simulink model "bus_as_currentsource_charging_discharging_battery_1"  (R2023a)
settings: Solver=VariableStepAuto  StartTime=0.0  StopTime=0.01  RelTol=1e-3
libraries: spsParallelRLCBranchLib x72, spsCurrentMeasurementLib x27, spsVoltageMeasurementLib x27, spspowerguiLib x25, spsControlledVoltageSourceLib x24, spsVariableResistorLib x24, spsSeriesRLCBranchLib x6, spsMosfetLib x2, sdolib x1, spsControlledCurrentSourceLib x1, spsGroundLib x1
(part 1 of 4)
settings Model: Creator=mluser  LastModifiedBy=Amith

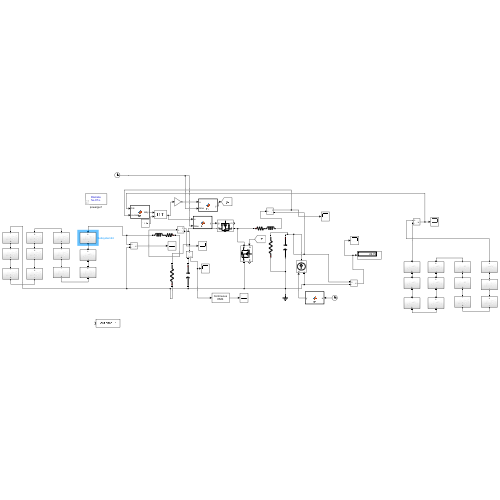
[thumbnail: Simulink's stored preview of the top-level diagram]
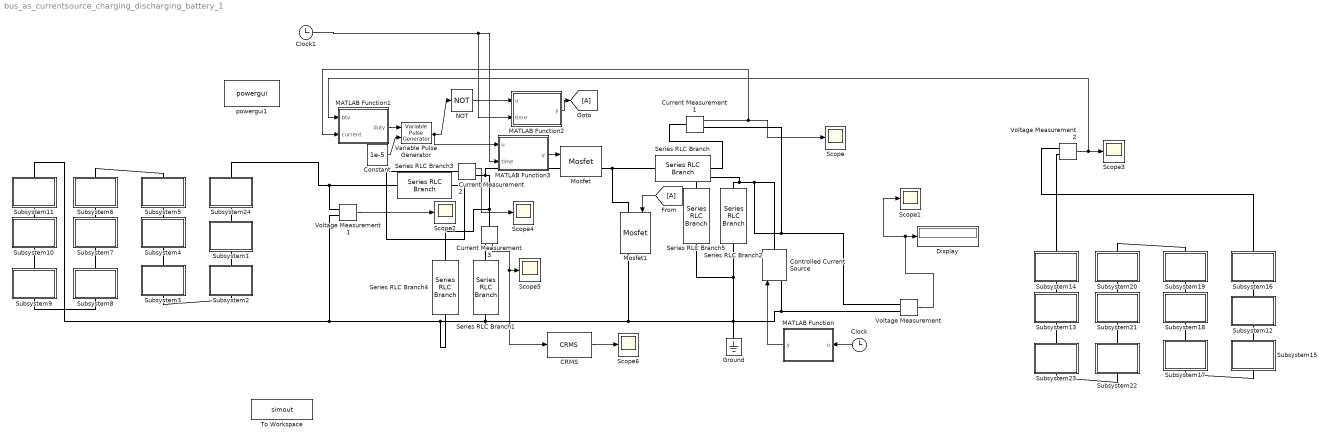
== system bus_as_currentsource_charging_discharging_battery_1 ==
  CRMS : sdolib/RMS Blocks/CRMS
  Clock : Clock
  Clock1 : Clock
  Constant : Constant  Value=1e-5
  Controlled Current Source : spsControlledCurrentSourceLib/Controlled Current Source  Initialize=on  Source_Type=AC  Amplitude=0  Phase=0  Frequency=0  Measurements=None
  Current Measurement1 : spsCurrentMeasurementLib/Current Measurement  PhasorSimulation=off  OutputType=Complex  PSBequivalent=0
  Current Measurement2 : spsCurrentMeasurementLib/Current Measurement  PhasorSimulation=off  OutputType=Complex  PSBequivalent=0
  Current Measurement3 : spsCurrentMeasurementLib/Current Measurement  PhasorSimulation=off  OutputType=Complex  PSBequivalent=0
  Display : Display
  From : From
  Goto : Goto
  Ground : spsGroundLib/Ground  LConnTagsString=a
  MATLAB Function : MATLAB Function  TreatAsAtomicUnit=on
  MATLAB Function1 : MATLAB Function  TreatAsAtomicUnit=on
  MATLAB Function2 : MATLAB Function  TreatAsAtomicUnit=on
  MATLAB Function3 : MATLAB Function  TreatAsAtomicUnit=on
  Mosfet : spsMosfetLib/Mosfet  Ron=0.1  Lon=0  Rd=0.01  Vfd=0  IC=0  Rs=1e5  Cs=inf  Measurements=on
  Mosfet1 : spsMosfetLib/Mosfet  Ron=0.1  Lon=0  Rd=0.01  Vfd=0  IC=0  Rs=1e5  Cs=inf  Measurements=on
  NOT : Logic  Operator=NOT  IconShape=distinctive  AllPortsSameDT=off  OutDataTypeStr=boolean
  Scope{,1..6} (7 alike) : Scope
  Series RLC Branch : spsSeriesRLCBranchLib/Series RLC Branch  LConnTagsString=__new0  RConnTagsString=__new0  BranchType=RL  Resistance=2.4e-3  Inductance=22e-6  SetiL0=off  InitialCurrent=0  Capacitance=1e-6  Setx0=off  InitialVoltage=0  Measurements=None
  Series RLC Branch1 : spsSeriesRLCBranchLib/Series RLC Branch  LConnTagsString=__new0  RConnTagsString=__new0  BranchType=C  Resistance=1  Inductance=1e-3  SetiL0=off  InitialCurrent=0  Capacitance=94e-6  Setx0=off  InitialVoltage=0  Measurements=None
  Series RLC Branch2 : spsSeriesRLCBranchLib/Series RLC Branch  LConnTagsString=__new0  RConnTagsString=__new0  BranchType=C  Resistance=1  Inductance=1e-3  SetiL0=off  InitialCurrent=0  Capacitance=188e-6  Setx0=off  InitialVoltage=0  Measurements=None
  Series RLC Branch3 : spsSeriesRLCBranchLib/Series RLC Branch  LConnTagsString=__new0  RConnTagsString=__new0  BranchType=RL  Resistance=2.4e-3  Inductance=22e-6  SetiL0=off  InitialCurrent=0  Capacitance=256.86e-6  Setx0=off  InitialVoltage=0  Measurements=None
  Series RLC Branch4 : spsSeriesRLCBranchLib/Series RLC Branch  LConnTagsString=__new0  RConnTagsString=__new0  BranchType=R  Resistance=10e3  Inductance=22e-6  SetiL0=off  InitialCurrent=0  Capacitance=256.86e-6  Setx0=off  InitialVoltage=0  Measurements=None
  Series RLC Branch5 : spsSeriesRLCBranchLib/Series RLC Branch  LConnTagsString=__new0  RConnTagsString=__new0  BranchType=R  Resistance=10e3  Inductance=22e-6  SetiL0=off  InitialCurrent=0  Capacitance=256.86e-6  Setx0=off  InitialVoltage=0  Measurements=None
  Subsystem1 : Subsystem
  Subsystem10 : Subsystem
  Subsystem11 : Subsystem
  Subsystem12 : Subsystem
  Subsystem13 : Subsystem
  Subsystem14 : Subsystem
  Subsystem15 : Subsystem
  Subsystem16 : Subsystem
  Subsystem17 : Subsystem
  Subsystem18 : Subsystem
  Subsystem19 : Subsystem
  Subsystem2 : Subsystem
  Subsystem20 : Subsystem
  Subsystem21 : Subsystem
  Subsystem22 : Subsystem
  Subsystem23 : Subsystem
  Subsystem24 : Subsystem
  Subsystem3 : Subsystem
  Subsystem4 : Subsystem
  Subsystem5 : Subsystem
  Subsystem6 : Subsystem
  Subsystem7 : Subsystem
  Subsystem8 : Subsystem
  Subsystem9 : Subsystem
  To Workspace : ToWorkspace  VariableName=simout  SaveFormat=Timeseries  SampleTime=-1
  Variable Pulse Generator : VariablePulseGenerator  SampleTime=0.1
  Voltage Measurement : spsVoltageMeasurementLib/Voltage Measurement  PhasorSimulation=off  OutputType=Complex  PSBequivalent=0
  Voltage Measurement1 : spsVoltageMeasurementLib/Voltage Measurement  PhasorSimulation=off  OutputType=Complex  PSBequivalent=0
  Voltage Measurement2 : spsVoltageMeasurementLib/Voltage Measurement  PhasorSimulation=off  OutputType=Complex  PSBequivalent=0
  powergui1 : spspowerguiLib/powergui  Priority=1  SimulationMode=Discrete  SampleTime=5e-7  frequency=60  Iterations=50  frequencyindice=0  Pbase=100e6  ErrMax=1e-4  UnitsV=kV  UnitsW=MW  buscounter=0  FunctionMessages=off  echomessages=off  EnableUseOfTLC=off  CurrentSourceSwitches=off  DisableSnubberDevices=off  DisableRonSwitches=off  DisableVfSwitches=off  DisplayEquations=off  AutomaticDiscreteSolvers=off  SolverType=Tustin/Backward Euler (TBE)  Interpol=off  ExternalGateDelay=off  methode=off  Ts=100  x0status=blocks  SPID=on  SwTol=0  HookPort=off  NonlinearTolerance=1e-4  nMaxIteration=100  ContinueOnMaxIteration=off  RestoreLinks=warning  ResistiveCurrentMeasurement=off  Frange=[0:2:500]  Ylog=off  Xlog=on  ShowGrid=off  save=off  variable=ZData  structure=0  ZoomFFT=off  StartTime=0.0  cycles=1  DisplayStyle=1  fundamental=60  FreqAxis=off  MaxFrequency=1000  frequencyindicesteady=1  RmsSteady=1  display=off
  wires:
  Clock1/1 -> MATLAB Function3/2(time), MATLAB Function2/2(time)
  Variable Pulse Generator/1 -> MATLAB Function3/1(u), NOT/1
  MATLAB Function1/1(duty) -> Variable Pulse Generator/1
  Current Measurement2/1 -> Scope4/1
  MATLAB Function/1(y) -> Controlled Current Source/1
  MATLAB Function3/1(y) -> Mosfet/1
  From/1 -> Mosfet1/1
  Voltage Measurement1/1 -> Scope2/1
  Clock/1 -> MATLAB Function/1(u)
  NOT/1 -> MATLAB Function2/1(u)
  Voltage Measurement2/1 -> MATLAB Function1/1(btv), Scope3/1
  Current Measurement1/1 -> MATLAB Function1/2(current), Scope/1
  MATLAB Function2/1(y) -> Goto/1
  Current Measurement3/1 -> CRMS/1, Scope5/1
  Constant/1 -> Variable Pulse Generator/2
  Voltage Measurement/1 -> Scope1/1, Display/1
  CRMS/1 -> Scope6/1
  connections:
  Mosfet/LConn1 -- Current Measurement2/RConn1 -- Series RLC Branch4/RConn1 -- Current Measurement3/LConn1
  Voltage Measurement/LConn2 -- Ground/LConn1 -- Series RLC Branch5/LConn1 -- Series RLC Branch2/RConn1 -- Subsystem11/LConn1 -- Voltage Measurement1/LConn2 -- Series RLC Branch4/LConn1 -- Series RLC Branch1/RConn1 -- Mosfet1/RConn1 -- Controlled Current Source/LConn1
  Voltage Measurement/LConn1 -- Controlled Current Source/RConn1 -- Series RLC Branch5/RConn1 -- Series RLC Branch2/LConn1 -- Current Measurement1/RConn1
  Mosfet1/LConn1 -- Series RLC Branch/LConn1 -- Mosfet/RConn1
  Voltage Measurement1/LConn1 -- Subsystem24/RConn1 -- Series RLC Branch3/RConn1
  Series RLC Branch1/LConn1 -- Current Measurement3/RConn1
  Current Measurement2/LConn1 -- Series RLC Branch3/LConn1
  Current Measurement1/LConn1 -- Series RLC Branch/RConn1
  Subsystem1/RConn1 -- Subsystem24/LConn1
  Subsystem2/RConn1 -- Subsystem1/LConn1
  Subsystem3/RConn1 -- Subsystem2/LConn1
  Subsystem6/RConn1 -- Subsystem5/LConn1
  Subsystem5/RConn1 -- Subsystem4/LConn1
  Subsystem10/RConn1 -- Subsystem9/LConn1
  Subsystem4/RConn1 -- Subsystem3/LConn1
  Subsystem7/RConn1 -- Subsystem6/LConn1
  Subsystem8/LConn1 -- Subsystem9/RConn1
  Subsystem11/RConn1 -- Subsystem10/LConn1
  Subsystem8/RConn1 -- Subsystem7/LConn1
  Subsystem12/RConn1 -- Subsystem16/LConn1
  Subsystem22/RConn1 -- Subsystem21/LConn1
  Subsystem20/RConn1 -- Subsystem19/LConn1
  Subsystem14/RConn1 -- Subsystem13/LConn1
  Subsystem21/RConn1 -- Subsystem20/LConn1
  Subsystem15/RConn1 -- Subsystem12/LConn1
  Subsystem19/RConn1 -- Subsystem18/LConn1
  Subsystem13/RConn1 -- Subsystem23/LConn1
  Subsystem18/RConn1 -- Subsystem17/LConn1
  Subsystem14/LConn1 -- Voltage Measurement2/LConn2
  Subsystem16/RConn1 -- Voltage Measurement2/LConn1
  Subsystem15/LConn1 -- Subsystem17/RConn1
  Subsystem22/LConn1 -- Subsystem23/RConn1

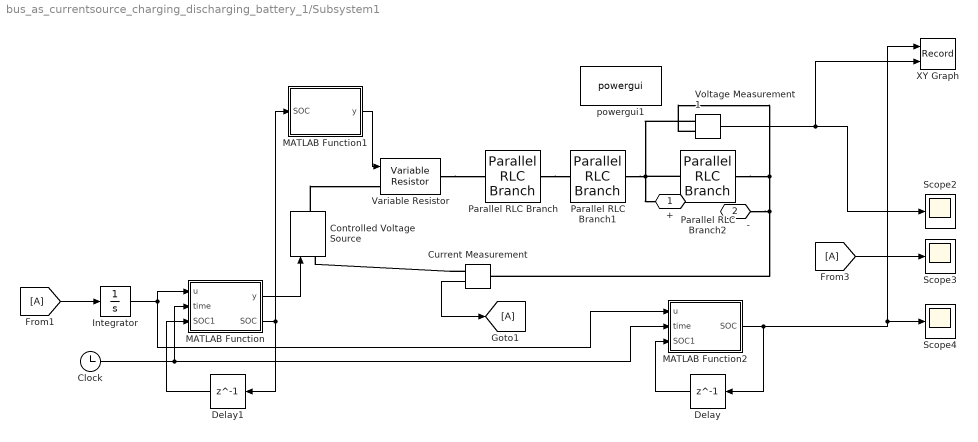
== system bus_as_currentsource_charging_discharging_battery_1/Subsystem1 ==
  Clock : Clock
  Controlled Voltage Source : spsControlledVoltageSourceLib/Controlled Voltage Source  Initialize=on  Source_Type=DC  Amplitude=0  Phase=0  Frequency=0  Measurements=None
  Current Measurement : spsCurrentMeasurementLib/Current Measurement  PhasorSimulation=off  OutputType=Complex  PSBequivalent=0
  Delay : Delay  DelayLength=1  InitialCondition=0
  Delay1 : Delay  DelayLength=1  InitialCondition=0
  From1 : From
  From3 : From
  Goto1 : Goto
  Integrator : Integrator
  MATLAB Function : MATLAB Function  TreatAsAtomicUnit=on
  MATLAB Function1 : MATLAB Function  TreatAsAtomicUnit=on
  MATLAB Function2 : MATLAB Function  TreatAsAtomicUnit=on
  Parallel RLC Branch : spsParallelRLCBranchLib/Parallel RLC Branch  LConnTagsString=a  RConnTagsString=__new0  BranchType=RC  Resistance=15.5e-3  Inductance=1e-3  SetiL0=off  InitialCurrent=0  Capacitance=1028.7  Setx0=off  InitialVoltage=0  Measurements=None
  Parallel RLC Branch1 : spsParallelRLCBranchLib/Parallel RLC Branch  LConnTagsString=a  RConnTagsString=__new0  BranchType=RC  Resistance=18.3e-3  Inductance=1e-3  SetiL0=off  InitialCurrent=0  Capacitance=5756.6  Setx0=off  InitialVoltage=0  Measurements=None
  Parallel RLC Branch2 : spsParallelRLCBranchLib/Parallel RLC Branch  LConnTagsString=a  RConnTagsString=__new0  BranchType=R  Resistance=1e9  Inductance=1e-3  SetiL0=off  InitialCurrent=0  Capacitance=5756.6  Setx0=off  InitialVoltage=0  Measurements=None
  Scope2 : Scope
  Scope3 : Scope
  Scope4 : Scope
  Variable Resistor : spsVariableResistorLib/Variable Resistor  Rabsmin=1e-3
      settings: LibrarySourceBlock=sps_lib/Passives/Variable Resistor
  Voltage Measurement1 : spsVoltageMeasurementLib/Voltage Measurement  PhasorSimulation=off  OutputType=Complex  PSBequivalent=0
  XY Graph : Record  FileSettingsInternal="{\"entries\":[{\"content\":{\"excelSettings\":{\"content\":{},\"type\":\"Streamout.ExcelSettings\"}},\"type\":\"Streamout.FileSettingStorage\",\"uuid\":\"4061d31d-d8a3-4fd0-9d33-75a5776b2999\"}],\"packageUris\":[\"http://schema.mathworks.com/mf0/streamout_blocks/R2020a\"],\"version\":\"1.0\"}"  Layout=[1 1]  SignalsInternal="{\"entries\":[{\"content\":{\"signals\":[{\"content\":{\"blockPath\":[\"bus_as_currentsource_charging_discharging_battery_1/Subsystem1/XY Graph\"],\"dimensions\":[1],\"domain\":\"bus_as_currentsource_charging_discharging_battery_1/Subsystem1/XY Graph\",\"lineColor\":\"#a2142f\",\"port\":1,\"sid\":[\"\"],\"signalID\":203,\"signalName\":\"MATLAB Function2\"},\"type\":\"RecordBlkView.Signal\",\"uuid\":\"0f566fc9-80d1-47d5-bf49-5749430e9d0a\"},{\"content\":{\"blockPath\":[\"bus_as_currentsource_charging_discharging_battery_1/Subsystem1/XY Graph\"],\"dimensions\":[1],\"domain\":\"bus_as_currentsource_charging_discharging_battery_1/Subsystem1/XY Graph\",\"lineColor\":\"#139fff\",\"port\":2,\"sid\":[\"\"],\"signalID\":207,\"signalName\":\"Voltage Measurement1\"},\"type\":\"RecordBlkView.Signal\",\"uuid\":\"ed6d931e-a948-4cdc-a839-bfb3bbb69890\"}]},\"type\":\"RecordBlkView.InputSignals\",\"uuid\":\"04ab3669-a145-4f40-a759-cdf575706550\"}],\"packageUris\":[\"http://schema.mathworks.com/mf0/streamout_blocks/R2020a\"],\"version\":\"1.0\"}"  VisualizationBindings="{\"xyplotplugin\":{\"info\":[{\"series\":[],\"subplotID\":1}]}}"  CompatibilityTag=XY
  powergui1 : spspowerguiLib/powergui  Priority=1  SimulationMode=Discrete  SampleTime=2e-7  frequency=60  Iterations=50  frequencyindice=0  Pbase=100e6  ErrMax=1e-4  UnitsV=kV  UnitsW=MW  buscounter=0  FunctionMessages=off  echomessages=off  EnableUseOfTLC=off  CurrentSourceSwitches=off  DisableSnubberDevices=off  DisableRonSwitches=off  DisableVfSwitches=off  DisplayEquations=off  AutomaticDiscreteSolvers=off  SolverType=Tustin/Backward Euler (TBE)  Interpol=off  ExternalGateDelay=off  methode=off  Ts=100  x0status=blocks  SPID=on  SwTol=0  HookPort=off  NonlinearTolerance=1e-4  nMaxIteration=100  ContinueOnMaxIteration=off  RestoreLinks=warning  ResistiveCurrentMeasurement=off  Frange=[0:2:500]  Ylog=off  Xlog=on  ShowGrid=off  save=off  variable=ZData  structure=0  ZoomFFT=off  StartTime=0.0  cycles=1  DisplayStyle=1  fundamental=60  FreqAxis=off  MaxFrequency=1000  frequencyindicesteady=1  RmsSteady=1  display=off
  + : PMIOPort  Side=Right
  - : PMIOPort  Port=2  Side=Left
  wires:
  Current Measurement/1 -> Goto1/1
  From3/1 -> Scope3/1
  Voltage Measurement1/1 -> XY Graph/2, Scope2/1
  MATLAB Function2/1(SOC) -> Delay/1, XY Graph/1, Scope4/1
  From1/1 -> Integrator/1
  MATLAB Function/1(y) -> Controlled Voltage Source/1
  MATLAB Function1/1(y) -> Variable Resistor/1
  Integrator/1 -> MATLAB Function2/1(u), MATLAB Function/1(u)
  Clock/1 -> MATLAB Function2/2(time), MATLAB Function/2(time)
  MATLAB Function/2(SOC) -> Delay1/1, MATLAB Function1/1(SOC)
  Delay/1 -> MATLAB Function2/3(SOC1)
  Delay1/1 -> MATLAB Function/3(SOC1)
  connections:
  Variable Resistor/RConn1 -- Parallel RLC Branch/LConn1
  Parallel RLC Branch1/RConn1 -- Parallel RLC Branch2/LConn1 -- +/RConn1 -- Voltage Measurement1/LConn1
  Voltage Measurement1/LConn2 -- Parallel RLC Branch2/RConn1 -- -/RConn1 -- Current Measurement/LConn1
  Controlled Voltage Source/RConn1 -- Variable Resistor/LConn1
  Current Measurement/RConn1 -- Controlled Voltage Source/LConn1
  Parallel RLC Branch/RConn1 -- Parallel RLC Branch1/LConn1

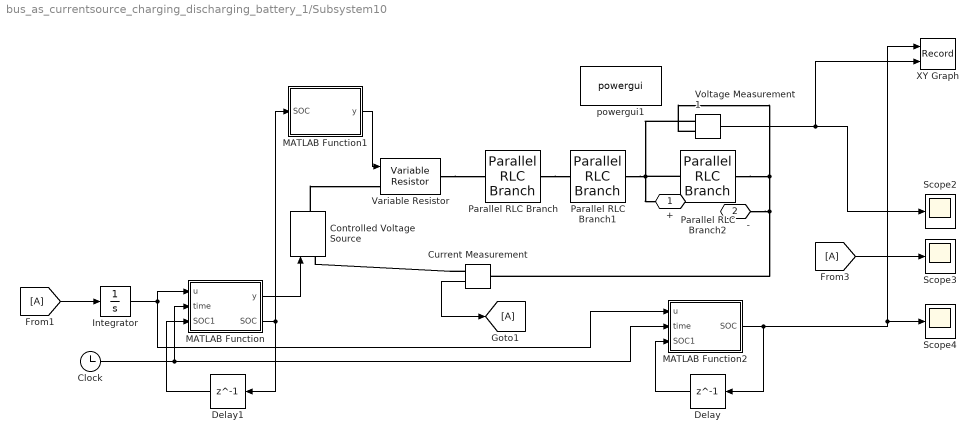
== system bus_as_currentsource_charging_discharging_battery_1/Subsystem10 ==
  Clock : Clock
  Controlled Voltage Source : spsControlledVoltageSourceLib/Controlled Voltage Source  Initialize=on  Source_Type=DC  Amplitude=0  Phase=0  Frequency=0  Measurements=None
  Current Measurement : spsCurrentMeasurementLib/Current Measurement  PhasorSimulation=off  OutputType=Complex  PSBequivalent=0
  Delay : Delay  DelayLength=1  InitialCondition=0
  Delay1 : Delay  DelayLength=1  InitialCondition=0
  From1 : From
  From3 : From
  Goto1 : Goto
  Integrator : Integrator
  MATLAB Function : MATLAB Function  TreatAsAtomicUnit=on
  MATLAB Function1 : MATLAB Function  TreatAsAtomicUnit=on
  MATLAB Function2 : MATLAB Function  TreatAsAtomicUnit=on
  Parallel RLC Branch : spsParallelRLCBranchLib/Parallel RLC Branch  LConnTagsString=a  RConnTagsString=__new0  BranchType=RC  Resistance=15.5e-3  Inductance=1e-3  SetiL0=off  InitialCurrent=0  Capacitance=1028.7  Setx0=off  InitialVoltage=0  Measurements=None
  Parallel RLC Branch1 : spsParallelRLCBranchLib/Parallel RLC Branch  LConnTagsString=a  RConnTagsString=__new0  BranchType=RC  Resistance=18.3e-3  Inductance=1e-3  SetiL0=off  InitialCurrent=0  Capacitance=5756.6  Setx0=off  InitialVoltage=0  Measurements=None
  Parallel RLC Branch2 : spsParallelRLCBranchLib/Parallel RLC Branch  LConnTagsString=a  RConnTagsString=__new0  BranchType=R  Resistance=1e9  Inductance=1e-3  SetiL0=off  InitialCurrent=0  Capacitance=5756.6  Setx0=off  InitialVoltage=0  Measurements=None
  Scope2 : Scope
  Scope3 : Scope
  Scope4 : Scope
  Variable Resistor : spsVariableResistorLib/Variable Resistor  Rabsmin=1e-3
      settings: LibrarySourceBlock=sps_lib/Passives/Variable Resistor
  Voltage Measurement1 : spsVoltageMeasurementLib/Voltage Measurement  PhasorSimulation=off  OutputType=Complex  PSBequivalent=0
  XY Graph : Record  FileSettingsInternal="{\"entries\":[{\"content\":{\"excelSettings\":{\"content\":{},\"type\":\"Streamout.ExcelSettings\"}},\"type\":\"Streamout.FileSettingStorage\",\"uuid\":\"1acef1d3-1533-4111-95e4-15d755019280\"}],\"packageUris\":[\"http://schema.mathworks.com/mf0/streamout_blocks/R2020a\"],\"version\":\"1.0\"}"  Layout=[1 1]  SignalsInternal="{\"entries\":[{\"content\":{\"signals\":[{\"content\":{\"blockPath\":[\"bus_as_currentsource_charging_discharging_battery_1/Subsystem10/XY Graph\"],\"dimensions\":[1],\"domain\":\"bus_as_currentsource_charging_discharging_battery_1/Subsystem10/XY Graph\",\"lineColor\":\"#ff6929\",\"port\":1,\"sid\":[\"\"],\"signalID\":211,\"signalName\":\"MATLAB Function2\"},\"type\":\"RecordBlkView.Signal\",\"uuid\":\"1c5f61ff-3524-492e-ac01-ee5e6fde95d9\"},{\"content\":{\"blockPath\":[\"bus_as_currentsource_charging_discharging_battery_1/Subsystem10/XY Graph\"],\"dimensions\":[1],\"domain\":\"bus_as_currentsource_charging_discharging_battery_1/Subsystem10/XY Graph\",\"lineColor\":\"#b746ff\",\"port\":2,\"sid\":[\"\"],\"signalID\":215,\"signalName\":\"Voltage Measurement1\"},\"type\":\"RecordBlkView.Signal\",\"uuid\":\"4a662dbb-6ada-419c-879e-f8766603ed58\"}]},\"type\":\"RecordBlkView.InputSignals\",\"uuid\":\"1ce9e898-f152-4a36-91f2-a929c2b13ee4\"}],\"packageUris\":[\"http://schema.mathworks.com/mf0/streamout_blocks/R2020a\"],\"version\":\"1.0\"}"  VisualizationBindings="{\"xyplotplugin\":{\"info\":[{\"series\":[],\"subplotID\":1}]}}"  CompatibilityTag=XY
  powergui1 : spspowerguiLib/powergui  Priority=1  SimulationMode=Discrete  SampleTime=2e-7  frequency=60  Iterations=50  frequencyindice=0  Pbase=100e6  ErrMax=1e-4  UnitsV=kV  UnitsW=MW  buscounter=0  FunctionMessages=off  echomessages=off  EnableUseOfTLC=off  CurrentSourceSwitches=off  DisableSnubberDevices=off  DisableRonSwitches=off  DisableVfSwitches=off  DisplayEquations=off  AutomaticDiscreteSolvers=off  SolverType=Tustin/Backward Euler (TBE)  Interpol=off  ExternalGateDelay=off  methode=off  Ts=100  x0status=blocks  SPID=on  SwTol=0  HookPort=off  NonlinearTolerance=1e-4  nMaxIteration=100  ContinueOnMaxIteration=off  RestoreLinks=warning  ResistiveCurrentMeasurement=off  Frange=[0:2:500]  Ylog=off  Xlog=on  ShowGrid=off  save=off  variable=ZData  structure=0  ZoomFFT=off  StartTime=0.0  cycles=1  DisplayStyle=1  fundamental=60  FreqAxis=off  MaxFrequency=1000  frequencyindicesteady=1  RmsSteady=1  display=off
  + : PMIOPort  Side=Right
  - : PMIOPort  Port=2  Side=Left
  wires:
  Current Measurement/1 -> Goto1/1
  From3/1 -> Scope3/1
  Voltage Measurement1/1 -> XY Graph/2, Scope2/1
  MATLAB Function2/1(SOC) -> Delay/1, XY Graph/1, Scope4/1
  From1/1 -> Integrator/1
  MATLAB Function/1(y) -> Controlled Voltage Source/1
  MATLAB Function1/1(y) -> Variable Resistor/1
  Integrator/1 -> MATLAB Function2/1(u), MATLAB Function/1(u)
  Clock/1 -> MATLAB Function2/2(time), MATLAB Function/2(time)
  MATLAB Function/2(SOC) -> Delay1/1, MATLAB Function1/1(SOC)
  Delay/1 -> MATLAB Function2/3(SOC1)
  Delay1/1 -> MATLAB Function/3(SOC1)
  connections:
  Variable Resistor/RConn1 -- Parallel RLC Branch/LConn1
  Parallel RLC Branch1/RConn1 -- Parallel RLC Branch2/LConn1 -- +/RConn1 -- Voltage Measurement1/LConn1
  Voltage Measurement1/LConn2 -- Parallel RLC Branch2/RConn1 -- -/RConn1 -- Current Measurement/LConn1
  Controlled Voltage Source/RConn1 -- Variable Resistor/LConn1
  Current Measurement/RConn1 -- Controlled Voltage Source/LConn1
  Parallel RLC Branch/RConn1 -- Parallel RLC Branch1/LConn1

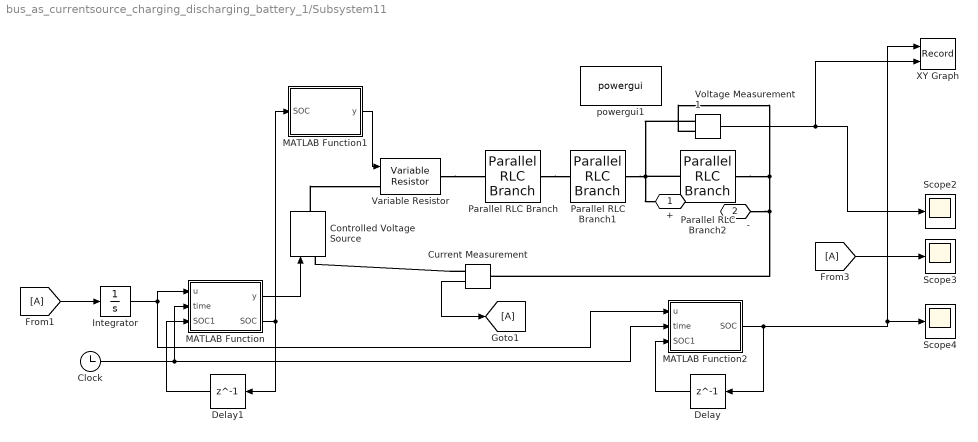
== system bus_as_currentsource_charging_discharging_battery_1/Subsystem11 ==
  Clock : Clock
  Controlled Voltage Source : spsControlledVoltageSourceLib/Controlled Voltage Source  Initialize=on  Source_Type=DC  Amplitude=0  Phase=0  Frequency=0  Measurements=None
  Current Measurement : spsCurrentMeasurementLib/Current Measurement  PhasorSimulation=off  OutputType=Complex  PSBequivalent=0
  Delay : Delay  DelayLength=1  InitialCondition=0
  Delay1 : Delay  DelayLength=1  InitialCondition=0
  From1 : From
  From3 : From
  Goto1 : Goto
  Integrator : Integrator
  MATLAB Function : MATLAB Function  TreatAsAtomicUnit=on
  MATLAB Function1 : MATLAB Function  TreatAsAtomicUnit=on
  MATLAB Function2 : MATLAB Function  TreatAsAtomicUnit=on
  Parallel RLC Branch : spsParallelRLCBranchLib/Parallel RLC Branch  LConnTagsString=a  RConnTagsString=__new0  BranchType=RC  Resistance=15.5e-3  Inductance=1e-3  SetiL0=off  InitialCurrent=0  Capacitance=1028.7  Setx0=off  InitialVoltage=0  Measurements=None
  Parallel RLC Branch1 : spsParallelRLCBranchLib/Parallel RLC Branch  LConnTagsString=a  RConnTagsString=__new0  BranchType=RC  Resistance=18.3e-3  Inductance=1e-3  SetiL0=off  InitialCurrent=0  Capacitance=5756.6  Setx0=off  InitialVoltage=0  Measurements=None
  Parallel RLC Branch2 : spsParallelRLCBranchLib/Parallel RLC Branch  LConnTagsString=a  RConnTagsString=__new0  BranchType=R  Resistance=1e9  Inductance=1e-3  SetiL0=off  InitialCurrent=0  Capacitance=5756.6  Setx0=off  InitialVoltage=0  Measurements=None
  Scope2 : Scope
  Scope3 : Scope
  Scope4 : Scope
  Variable Resistor : spsVariableResistorLib/Variable Resistor  Rabsmin=1e-3
      settings: LibrarySourceBlock=sps_lib/Passives/Variable Resistor
  Voltage Measurement1 : spsVoltageMeasurementLib/Voltage Measurement  PhasorSimulation=off  OutputType=Complex  PSBequivalent=0
  XY Graph : Record  FileSettingsInternal="{\"entries\":[{\"content\":{\"excelSettings\":{\"content\":{},\"type\":\"Streamout.ExcelSettings\"}},\"type\":\"Streamout.FileSettingStorage\",\"uuid\":\"8663ecc0-cb66-412b-8c7b-e72bd5036c19\"}],\"packageUris\":[\"http://schema.mathworks.com/mf0/streamout_blocks/R2020a\"],\"version\":\"1.0\"}"  Layout=[1 1]  SignalsInternal="{\"entries\":[{\"content\":{\"signals\":[{\"content\":{\"blockPath\":[\"bus_as_currentsource_charging_discharging_battery_1/Subsystem11/XY Graph\"],\"dimensions\":[1],\"domain\":\"bus_as_currentsource_charging_discharging_battery_1/Subsystem11/XY Graph\",\"lineColor\":\"#64d413\",\"port\":1,\"sid\":[\"\"],\"signalID\":219,\"signalName\":\"MATLAB Function2\"},\"type\":\"RecordBlkView.Signal\",\"uuid\":\"0330ed62-72d8-4139-974a-3bd9369839bd\"},{\"content\":{\"blockPath\":[\"bus_as_currentsource_charging_discharging_battery_1/Subsystem11/XY Graph\"],\"dimensions\":[1],\"domain\":\"bus_as_currentsource_charging_discharging_battery_1/Subsystem11/XY Graph\",\"lineColor\":\"#ff13a6\",\"port\":2,\"sid\":[\"\"],\"signalID\":223,\"signalName\":\"Voltage Measurement1\"},\"type\":\"RecordBlkView.Signal\",\"uuid\":\"fdbe943a-62ce-4f49-b938-f7a2a0a2a25f\"}]},\"type\":\"RecordBlkView.InputSignals\",\"uuid\":\"49257015-2782-4ba8-a6e2-e68c29dc4fbc\"}],\"packageUris\":[\"http://schema.mathworks.com/mf0/streamout_blocks/R2020a\"],\"version\":\"1.0\"}"  VisualizationBindings="{\"xyplotplugin\":{\"info\":[{\"series\":[],\"subplotID\":1}]}}"  CompatibilityTag=XY
  powergui1 : spspowerguiLib/powergui  Priority=1  SimulationMode=Discrete  SampleTime=2e-7  frequency=60  Iterations=50  frequencyindice=0  Pbase=100e6  ErrMax=1e-4  UnitsV=kV  UnitsW=MW  buscounter=0  FunctionMessages=off  echomessages=off  EnableUseOfTLC=off  CurrentSourceSwitches=off  DisableSnubberDevices=off  DisableRonSwitches=off  DisableVfSwitches=off  DisplayEquations=off  AutomaticDiscreteSolvers=off  SolverType=Tustin/Backward Euler (TBE)  Interpol=off  ExternalGateDelay=off  methode=off  Ts=100  x0status=blocks  SPID=on  SwTol=0  HookPort=off  NonlinearTolerance=1e-4  nMaxIteration=100  ContinueOnMaxIteration=off  RestoreLinks=warning  ResistiveCurrentMeasurement=off  Frange=[0:2:500]  Ylog=off  Xlog=on  ShowGrid=off  save=off  variable=ZData  structure=0  ZoomFFT=off  StartTime=0.0  cycles=1  DisplayStyle=1  fundamental=60  FreqAxis=off  MaxFrequency=1000  frequencyindicesteady=1  RmsSteady=1  display=off
  + : PMIOPort  Side=Right
  - : PMIOPort  Port=2  Side=Left
  wires:
  Current Measurement/1 -> Goto1/1
  From3/1 -> Scope3/1
  Voltage Measurement1/1 -> XY Graph/2, Scope2/1
  MATLAB Function2/1(SOC) -> Delay/1, XY Graph/1, Scope4/1
  From1/1 -> Integrator/1
  MATLAB Function/1(y) -> Controlled Voltage Source/1
  MATLAB Function1/1(y) -> Variable Resistor/1
  Integrator/1 -> MATLAB Function2/1(u), MATLAB Function/1(u)
  Clock/1 -> MATLAB Function2/2(time), MATLAB Function/2(time)
  MATLAB Function/2(SOC) -> Delay1/1, MATLAB Function1/1(SOC)
  Delay/1 -> MATLAB Function2/3(SOC1)
  Delay1/1 -> MATLAB Function/3(SOC1)
  connections:
  Variable Resistor/RConn1 -- Parallel RLC Branch/LConn1
  Parallel RLC Branch1/RConn1 -- Parallel RLC Branch2/LConn1 -- +/RConn1 -- Voltage Measurement1/LConn1
  Voltage Measurement1/LConn2 -- Parallel RLC Branch2/RConn1 -- -/RConn1 -- Current Measurement/LConn1
  Controlled Voltage Source/RConn1 -- Variable Resistor/LConn1
  Current Measurement/RConn1 -- Controlled Voltage Source/LConn1
  Parallel RLC Branch/RConn1 -- Parallel RLC Branch1/LConn1

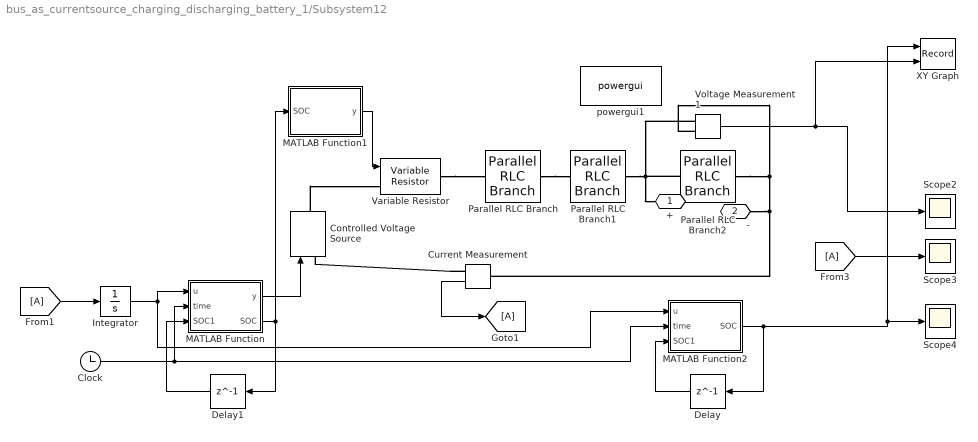
== system bus_as_currentsource_charging_discharging_battery_1/Subsystem12 ==
  Clock : Clock
  Controlled Voltage Source : spsControlledVoltageSourceLib/Controlled Voltage Source  Initialize=on  Source_Type=DC  Amplitude=0  Phase=0  Frequency=0  Measurements=None
  Current Measurement : spsCurrentMeasurementLib/Current Measurement  PhasorSimulation=off  OutputType=Complex  PSBequivalent=0
  Delay : Delay  DelayLength=1  InitialCondition=0
  Delay1 : Delay  DelayLength=1  InitialCondition=0
  From1 : From
  From3 : From
  Goto1 : Goto
  Integrator : Integrator
  MATLAB Function : MATLAB Function  TreatAsAtomicUnit=on
  MATLAB Function1 : MATLAB Function  TreatAsAtomicUnit=on
  MATLAB Function2 : MATLAB Function  TreatAsAtomicUnit=on
  Parallel RLC Branch : spsParallelRLCBranchLib/Parallel RLC Branch  LConnTagsString=a  RConnTagsString=__new0  BranchType=RC  Resistance=15.5e-3  Inductance=1e-3  SetiL0=off  InitialCurrent=0  Capacitance=1028.7  Setx0=off  InitialVoltage=0  Measurements=None
  Parallel RLC Branch1 : spsParallelRLCBranchLib/Parallel RLC Branch  LConnTagsString=a  RConnTagsString=__new0  BranchType=RC  Resistance=18.3e-3  Inductance=1e-3  SetiL0=off  InitialCurrent=0  Capacitance=5756.6  Setx0=off  InitialVoltage=0  Measurements=None
  Parallel RLC Branch2 : spsParallelRLCBranchLib/Parallel RLC Branch  LConnTagsString=a  RConnTagsString=__new0  BranchType=R  Resistance=1e9  Inductance=1e-3  SetiL0=off  InitialCurrent=0  Capacitance=5756.6  Setx0=off  InitialVoltage=0  Measurements=None
  Scope2 : Scope
  Scope3 : Scope
  Scope4 : Scope
  Variable Resistor : spsVariableResistorLib/Variable Resistor  Rabsmin=1e-3
      settings: LibrarySourceBlock=sps_lib/Passives/Variable Resistor
  Voltage Measurement1 : spsVoltageMeasurementLib/Voltage Measurement  PhasorSimulation=off  OutputType=Complex  PSBequivalent=0
  XY Graph : Record  FileSettingsInternal="{\"entries\":[{\"content\":{\"excelSettings\":{\"content\":{},\"type\":\"Streamout.ExcelSettings\"}},\"type\":\"Streamout.FileSettingStorage\",\"uuid\":\"e58bd3e6-da73-4c94-8daa-2e5cbd7139b3\"}],\"packageUris\":[\"http://schema.mathworks.com/mf0/streamout_blocks/R2020a\"],\"version\":\"1.0\"}"  Layout=[1 1]  SignalsInternal="{\"entries\":[{\"content\":{\"signals\":[{\"content\":{\"blockPath\":[\"bus_as_currentsource_charging_discharging_battery_1/Subsystem12/XY Graph\"],\"dimensions\":[1],\"domain\":\"bus_as_currentsource_charging_discharging_battery_1/Subsystem12/XY Graph\",\"lineColor\":\"#fe330a\",\"port\":1,\"sid\":[\"\"],\"signalID\":227,\"signalName\":\"MATLAB Function2\"},\"type\":\"RecordBlkView.Signal\",\"uuid\":\"194f4493-053b-448e-8ed1-f14f0cdefb82\"},{\"content\":{\"blockPath\":[\"bus_as_currentsource_charging_discharging_battery_1/Subsystem12/XY Graph\"],\"dimensions\":[1],\"domain\":\"bus_as_currentsource_charging_discharging_battery_1/Subsystem12/XY Graph\",\"lineColor\":\"#22b573\",\"port\":2,\"sid\":[\"\"],\"signalID\":231,\"signalName\":\"Voltage Measurement1\"},\"type\":\"RecordBlkView.Signal\",\"uuid\":\"fb7673e9-eb67-424c-972f-844387a5bd10\"}]},\"type\":\"RecordBlkView.InputSignals\",\"uuid\":\"4402b43d-c22b-4722-a95a-4f63b5b6fd7a\"}],\"packageUris\":[\"http://schema.mathworks.com/mf0/streamout_blocks/R2020a\"],\"version\":\"1.0\"}"  VisualizationBindings="{\"xyplotplugin\":{\"info\":[{\"series\":[],\"subplotID\":1}]}}"  CompatibilityTag=XY
  powergui1 : spspowerguiLib/powergui  Priority=1  SimulationMode=Discrete  SampleTime=2e-7  frequency=60  Iterations=50  frequencyindice=0  Pbase=100e6  ErrMax=1e-4  UnitsV=kV  UnitsW=MW  buscounter=0  FunctionMessages=off  echomessages=off  EnableUseOfTLC=off  CurrentSourceSwitches=off  DisableSnubberDevices=off  DisableRonSwitches=off  DisableVfSwitches=off  DisplayEquations=off  AutomaticDiscreteSolvers=off  SolverType=Tustin/Backward Euler (TBE)  Interpol=off  ExternalGateDelay=off  methode=off  Ts=100  x0status=blocks  SPID=on  SwTol=0  HookPort=off  NonlinearTolerance=1e-4  nMaxIteration=100  ContinueOnMaxIteration=off  RestoreLinks=warning  ResistiveCurrentMeasurement=off  Frange=[0:2:500]  Ylog=off  Xlog=on  ShowGrid=off  save=off  variable=ZData  structure=0  ZoomFFT=off  StartTime=0.0  cycles=1  DisplayStyle=1  fundamental=60  FreqAxis=off  MaxFrequency=1000  frequencyindicesteady=1  RmsSteady=1  display=off
  + : PMIOPort  Side=Right
  - : PMIOPort  Port=2  Side=Left
  wires:
  Current Measurement/1 -> Goto1/1
  From3/1 -> Scope3/1
  Voltage Measurement1/1 -> XY Graph/2, Scope2/1
  MATLAB Function2/1(SOC) -> Delay/1, XY Graph/1, Scope4/1
  From1/1 -> Integrator/1
  MATLAB Function/1(y) -> Controlled Voltage Source/1
  MATLAB Function1/1(y) -> Variable Resistor/1
  Integrator/1 -> MATLAB Function2/1(u), MATLAB Function/1(u)
  Clock/1 -> MATLAB Function2/2(time), MATLAB Function/2(time)
  MATLAB Function/2(SOC) -> Delay1/1, MATLAB Function1/1(SOC)
  Delay/1 -> MATLAB Function2/3(SOC1)
  Delay1/1 -> MATLAB Function/3(SOC1)
  connections:
  Variable Resistor/RConn1 -- Parallel RLC Branch/LConn1
  Parallel RLC Branch1/RConn1 -- Parallel RLC Branch2/LConn1 -- +/RConn1 -- Voltage Measurement1/LConn1
  Voltage Measurement1/LConn2 -- Parallel RLC Branch2/RConn1 -- -/RConn1 -- Current Measurement/LConn1
  Controlled Voltage Source/RConn1 -- Variable Resistor/LConn1
  Current Measurement/RConn1 -- Controlled Voltage Source/LConn1
  Parallel RLC Branch/RConn1 -- Parallel RLC Branch1/LConn1

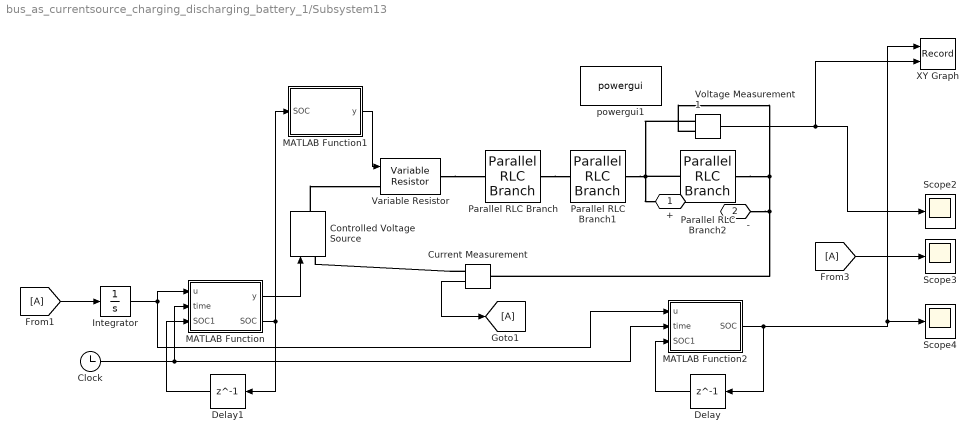
== system bus_as_currentsource_charging_discharging_battery_1/Subsystem13 ==
  Clock : Clock
  Controlled Voltage Source : spsControlledVoltageSourceLib/Controlled Voltage Source  Initialize=on  Source_Type=DC  Amplitude=0  Phase=0  Frequency=0  Measurements=None
  Current Measurement : spsCurrentMeasurementLib/Current Measurement  PhasorSimulation=off  OutputType=Complex  PSBequivalent=0
  Delay : Delay  DelayLength=1  InitialCondition=0
  Delay1 : Delay  DelayLength=1  InitialCondition=0
  From1 : From
  From3 : From
  Goto1 : Goto
  Integrator : Integrator
  MATLAB Function : MATLAB Function  TreatAsAtomicUnit=on
  MATLAB Function1 : MATLAB Function  TreatAsAtomicUnit=on
  MATLAB Function2 : MATLAB Function  TreatAsAtomicUnit=on
  Parallel RLC Branch : spsParallelRLCBranchLib/Parallel RLC Branch  LConnTagsString=a  RConnTagsString=__new0  BranchType=RC  Resistance=15.5e-3  Inductance=1e-3  SetiL0=off  InitialCurrent=0  Capacitance=1028.7  Setx0=off  InitialVoltage=0  Measurements=None
  Parallel RLC Branch1 : spsParallelRLCBranchLib/Parallel RLC Branch  LConnTagsString=a  RConnTagsString=__new0  BranchType=RC  Resistance=18.3e-3  Inductance=1e-3  SetiL0=off  InitialCurrent=0  Capacitance=5756.6  Setx0=off  InitialVoltage=0  Measurements=None
  Parallel RLC Branch2 : spsParallelRLCBranchLib/Parallel RLC Branch  LConnTagsString=a  RConnTagsString=__new0  BranchType=R  Resistance=1e9  Inductance=1e-3  SetiL0=off  InitialCurrent=0  Capacitance=5756.6  Setx0=off  InitialVoltage=0  Measurements=None
  Scope2 : Scope
  Scope3 : Scope
  Scope4 : Scope
  Variable Resistor : spsVariableResistorLib/Variable Resistor  Rabsmin=1e-3
      settings: LibrarySourceBlock=sps_lib/Passives/Variable Resistor
  Voltage Measurement1 : spsVoltageMeasurementLib/Voltage Measurement  PhasorSimulation=off  OutputType=Complex  PSBequivalent=0
  XY Graph : Record  FileSettingsInternal="{\"entries\":[{\"content\":{\"excelSettings\":{\"content\":{},\"type\":\"Streamout.ExcelSettings\"}},\"type\":\"Streamout.FileSettingStorage\",\"uuid\":\"8c4ec99f-2394-4e58-b599-ccdaa22fec52\"}],\"packageUris\":[\"http://schema.mathworks.com/mf0/streamout_blocks/R2020a\"],\"version\":\"1.0\"}"  Layout=[1 1]  SignalsInternal="{\"entries\":[{\"content\":{\"signals\":[{\"content\":{\"blockPath\":[\"bus_as_currentsource_charging_discharging_battery_1/Subsystem13/XY Graph\"],\"dimensions\":[1],\"domain\":\"bus_as_currentsource_charging_discharging_battery_1/Subsystem13/XY Graph\",\"lineColor\":\"#0072bd\",\"port\":1,\"sid\":[\"\"],\"signalID\":235,\"signalName\":\"MATLAB Function2\"},\"type\":\"RecordBlkView.Signal\",\"uuid\":\"9e83d846-9706-4b59-826d-6d5a7412411f\"},{\"content\":{\"blockPath\":[\"bus_as_currentsource_charging_discharging_battery_1/Subsystem13/XY Graph\"],\"dimensions\":[1],\"domain\":\"bus_as_currentsource_charging_discharging_battery_1/Subsystem13/XY Graph\",\"lineColor\":\"#d95319\",\"port\":2,\"sid\":[\"\"],\"signalID\":239,\"signalName\":\"Voltage Measurement1\"},\"type\":\"RecordBlkView.Signal\",\"uuid\":\"79db19ab-8b16-49cb-b752-70ca5c1f4ebc\"}]},\"type\":\"RecordBlkView.InputSignals\",\"uuid\":\"58da4e73-ddfd-4663-a45a-7ffeeb777d81\"}],\"packageUris\":[\"http://schema.mathworks.com/mf0/streamout_blocks/R2020a\"],\"version\":\"1.0\"}"  VisualizationBindings="{\"xyplotplugin\":{\"info\":[{\"series\":[],\"subplotID\":1}]}}"  CompatibilityTag=XY
  powergui1 : spspowerguiLib/powergui  Priority=1  SimulationMode=Discrete  SampleTime=2e-7  frequency=60  Iterations=50  frequencyindice=0  Pbase=100e6  ErrMax=1e-4  UnitsV=kV  UnitsW=MW  buscounter=0  FunctionMessages=off  echomessages=off  EnableUseOfTLC=off  CurrentSourceSwitches=off  DisableSnubberDevices=off  DisableRonSwitches=off  DisableVfSwitches=off  DisplayEquations=off  AutomaticDiscreteSolvers=off  SolverType=Tustin/Backward Euler (TBE)  Interpol=off  ExternalGateDelay=off  methode=off  Ts=100  x0status=blocks  SPID=on  SwTol=0  HookPort=off  NonlinearTolerance=1e-4  nMaxIteration=100  ContinueOnMaxIteration=off  RestoreLinks=warning  ResistiveCurrentMeasurement=off  Frange=[0:2:500]  Ylog=off  Xlog=on  ShowGrid=off  save=off  variable=ZData  structure=0  ZoomFFT=off  StartTime=0.0  cycles=1  DisplayStyle=1  fundamental=60  FreqAxis=off  MaxFrequency=1000  frequencyindicesteady=1  RmsSteady=1  display=off
  + : PMIOPort  Side=Right
  - : PMIOPort  Port=2  Side=Left
  wires:
  Current Measurement/1 -> Goto1/1
  From3/1 -> Scope3/1
  Voltage Measurement1/1 -> XY Graph/2, Scope2/1
  MATLAB Function2/1(SOC) -> Delay/1, XY Graph/1, Scope4/1
  From1/1 -> Integrator/1
  MATLAB Function/1(y) -> Controlled Voltage Source/1
  MATLAB Function1/1(y) -> Variable Resistor/1
  Integrator/1 -> MATLAB Function2/1(u), MATLAB Function/1(u)
  Clock/1 -> MATLAB Function2/2(time), MATLAB Function/2(time)
  MATLAB Function/2(SOC) -> Delay1/1, MATLAB Function1/1(SOC)
  Delay/1 -> MATLAB Function2/3(SOC1)
  Delay1/1 -> MATLAB Function/3(SOC1)
  connections:
  Variable Resistor/RConn1 -- Parallel RLC Branch/LConn1
  Parallel RLC Branch1/RConn1 -- Parallel RLC Branch2/LConn1 -- +/RConn1 -- Voltage Measurement1/LConn1
  Voltage Measurement1/LConn2 -- Parallel RLC Branch2/RConn1 -- -/RConn1 -- Current Measurement/LConn1
  Controlled Voltage Source/RConn1 -- Variable Resistor/LConn1
  Current Measurement/RConn1 -- Controlled Voltage Source/LConn1
  Parallel RLC Branch/RConn1 -- Parallel RLC Branch1/LConn1

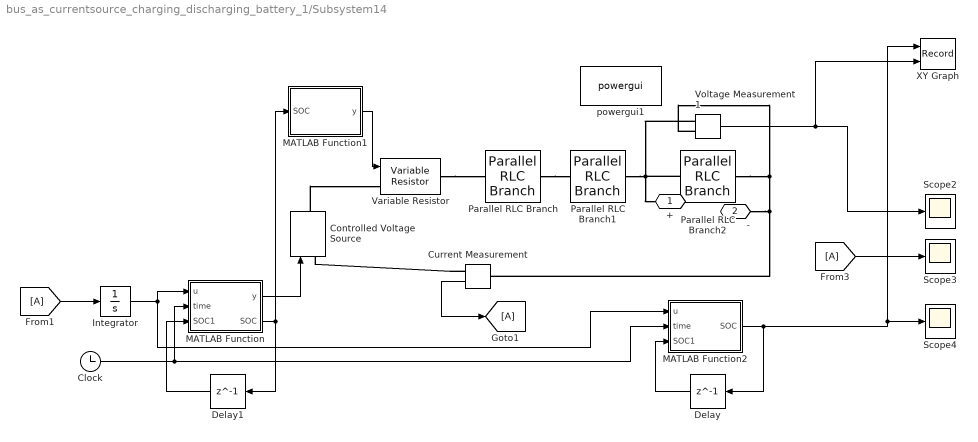
== system bus_as_currentsource_charging_discharging_battery_1/Subsystem14 ==
  Clock : Clock
  Controlled Voltage Source : spsControlledVoltageSourceLib/Controlled Voltage Source  Initialize=on  Source_Type=DC  Amplitude=0  Phase=0  Frequency=0  Measurements=None
  Current Measurement : spsCurrentMeasurementLib/Current Measurement  PhasorSimulation=off  OutputType=Complex  PSBequivalent=0
  Delay : Delay  DelayLength=1  InitialCondition=0
  Delay1 : Delay  DelayLength=1  InitialCondition=0
  From1 : From
  From3 : From
  Goto1 : Goto
  Integrator : Integrator
  MATLAB Function : MATLAB Function  TreatAsAtomicUnit=on
  MATLAB Function1 : MATLAB Function  TreatAsAtomicUnit=on
  MATLAB Function2 : MATLAB Function  TreatAsAtomicUnit=on
  Parallel RLC Branch : spsParallelRLCBranchLib/Parallel RLC Branch  LConnTagsString=a  RConnTagsString=__new0  BranchType=RC  Resistance=15.5e-3  Inductance=1e-3  SetiL0=off  InitialCurrent=0  Capacitance=1028.7  Setx0=off  InitialVoltage=0  Measurements=None
  Parallel RLC Branch1 : spsParallelRLCBranchLib/Parallel RLC Branch  LConnTagsString=a  RConnTagsString=__new0  BranchType=RC  Resistance=18.3e-3  Inductance=1e-3  SetiL0=off  InitialCurrent=0  Capacitance=5756.6  Setx0=off  InitialVoltage=0  Measurements=None
  Parallel RLC Branch2 : spsParallelRLCBranchLib/Parallel RLC Branch  LConnTagsString=a  RConnTagsString=__new0  BranchType=R  Resistance=1e9  Inductance=1e-3  SetiL0=off  InitialCurrent=0  Capacitance=5756.6  Setx0=off  InitialVoltage=0  Measurements=None
  Scope2 : Scope
  Scope3 : Scope
  Scope4 : Scope
  Variable Resistor : spsVariableResistorLib/Variable Resistor  Rabsmin=1e-3
      settings: LibrarySourceBlock=sps_lib/Passives/Variable Resistor
  Voltage Measurement1 : spsVoltageMeasurementLib/Voltage Measurement  PhasorSimulation=off  OutputType=Complex  PSBequivalent=0
  XY Graph : Record  FileSettingsInternal="{\"entries\":[{\"content\":{\"excelSettings\":{\"content\":{},\"type\":\"Streamout.ExcelSettings\"}},\"type\":\"Streamout.FileSettingStorage\",\"uuid\":\"83293d67-e47d-41a8-b344-5cdf4e3f8752\"}],\"packageUris\":[\"http://schema.mathworks.com/mf0/streamout_blocks/R2020a\"],\"version\":\"1.0\"}"  Layout=[1 1]  SignalsInternal="{\"entries\":[{\"content\":{\"signals\":[{\"content\":{\"blockPath\":[\"bus_as_currentsource_charging_discharging_battery_1/Subsystem14/XY Graph\"],\"dimensions\":[1],\"domain\":\"bus_as_currentsource_charging_discharging_battery_1/Subsystem14/XY Graph\",\"lineColor\":\"#edb120\",\"port\":1,\"sid\":[\"\"],\"signalID\":243,\"signalName\":\"MATLAB Function2\"},\"type\":\"RecordBlkView.Signal\",\"uuid\":\"d8673888-11c4-45fa-810f-6910e63b44bb\"},{\"content\":{\"blockPath\":[\"bus_as_currentsource_charging_discharging_battery_1/Subsystem14/XY Graph\"],\"dimensions\":[1],\"domain\":\"bus_as_currentsource_charging_discharging_battery_1/Subsystem14/XY Graph\",\"lineColor\":\"#7e2f8e\",\"port\":2,\"sid\":[\"\"],\"signalID\":247,\"signalName\":\"Voltage Measurement1\"},\"type\":\"RecordBlkView.Signal\",\"uuid\":\"cce21722-e92f-41a6-b892-bba42917ba4a\"}]},\"type\":\"RecordBlkView.InputSignals\",\"uuid\":\"21982cf0-558a-4000-97fe-662ea696ef32\"}],\"packageUris\":[\"http://schema.mathworks.com/mf0/streamout_blocks/R2020a\"],\"version\":\"1.0\"}"  VisualizationBindings="{\"xyplotplugin\":{\"info\":[{\"series\":[],\"subplotID\":1}]}}"  CompatibilityTag=XY
  powergui1 : spspowerguiLib/powergui  Priority=1  SimulationMode=Discrete  SampleTime=2e-7  frequency=60  Iterations=50  frequencyindice=0  Pbase=100e6  ErrMax=1e-4  UnitsV=kV  UnitsW=MW  buscounter=0  FunctionMessages=off  echomessages=off  EnableUseOfTLC=off  CurrentSourceSwitches=off  DisableSnubberDevices=off  DisableRonSwitches=off  DisableVfSwitches=off  DisplayEquations=off  AutomaticDiscreteSolvers=off  SolverType=Tustin/Backward Euler (TBE)  Interpol=off  ExternalGateDelay=off  methode=off  Ts=100  x0status=blocks  SPID=on  SwTol=0  HookPort=off  NonlinearTolerance=1e-4  nMaxIteration=100  ContinueOnMaxIteration=off  RestoreLinks=warning  ResistiveCurrentMeasurement=off  Frange=[0:2:500]  Ylog=off  Xlog=on  ShowGrid=off  save=off  variable=ZData  structure=0  ZoomFFT=off  StartTime=0.0  cycles=1  DisplayStyle=1  fundamental=60  FreqAxis=off  MaxFrequency=1000  frequencyindicesteady=1  RmsSteady=1  display=off
  + : PMIOPort  Side=Right
  - : PMIOPort  Port=2  Side=Left
  wires:
  Current Measurement/1 -> Goto1/1
  From3/1 -> Scope3/1
  Voltage Measurement1/1 -> XY Graph/2, Scope2/1
  MATLAB Function2/1(SOC) -> Delay/1, XY Graph/1, Scope4/1
  From1/1 -> Integrator/1
  MATLAB Function/1(y) -> Controlled Voltage Source/1
  MATLAB Function1/1(y) -> Variable Resistor/1
  Integrator/1 -> MATLAB Function2/1(u), MATLAB Function/1(u)
  Clock/1 -> MATLAB Function2/2(time), MATLAB Function/2(time)
  MATLAB Function/2(SOC) -> Delay1/1, MATLAB Function1/1(SOC)
  Delay/1 -> MATLAB Function2/3(SOC1)
  Delay1/1 -> MATLAB Function/3(SOC1)
  connections:
  Variable Resistor/RConn1 -- Parallel RLC Branch/LConn1
  Parallel RLC Branch1/RConn1 -- Parallel RLC Branch2/LConn1 -- +/RConn1 -- Voltage Measurement1/LConn1
  Voltage Measurement1/LConn2 -- Parallel RLC Branch2/RConn1 -- -/RConn1 -- Current Measurement/LConn1
  Controlled Voltage Source/RConn1 -- Variable Resistor/LConn1
  Current Measurement/RConn1 -- Controlled Voltage Source/LConn1
  Parallel RLC Branch/RConn1 -- Parallel RLC Branch1/LConn1

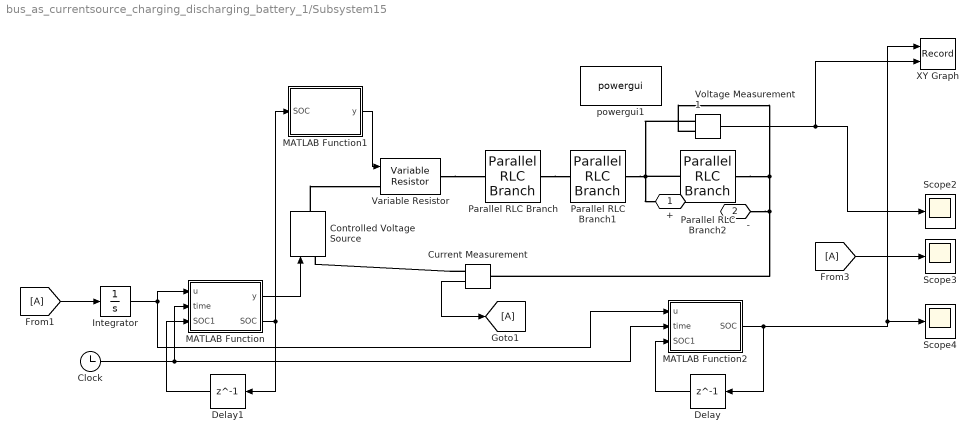
== system bus_as_currentsource_charging_discharging_battery_1/Subsystem15 ==
  Clock : Clock
  Controlled Voltage Source : spsControlledVoltageSourceLib/Controlled Voltage Source  Initialize=on  Source_Type=DC  Amplitude=0  Phase=0  Frequency=0  Measurements=None
  Current Measurement : spsCurrentMeasurementLib/Current Measurement  PhasorSimulation=off  OutputType=Complex  PSBequivalent=0
  Delay : Delay  DelayLength=1  InitialCondition=0
  Delay1 : Delay  DelayLength=1  InitialCondition=0
  From1 : From
  From3 : From
  Goto1 : Goto
  Integrator : Integrator
  MATLAB Function : MATLAB Function  TreatAsAtomicUnit=on
  MATLAB Function1 : MATLAB Function  TreatAsAtomicUnit=on
  MATLAB Function2 : MATLAB Function  TreatAsAtomicUnit=on
  Parallel RLC Branch : spsParallelRLCBranchLib/Parallel RLC Branch  LConnTagsString=a  RConnTagsString=__new0  BranchType=RC  Resistance=15.5e-3  Inductance=1e-3  SetiL0=off  InitialCurrent=0  Capacitance=1028.7  Setx0=off  InitialVoltage=0  Measurements=None
  Parallel RLC Branch1 : spsParallelRLCBranchLib/Parallel RLC Branch  LConnTagsString=a  RConnTagsString=__new0  BranchType=RC  Resistance=18.3e-3  Inductance=1e-3  SetiL0=off  InitialCurrent=0  Capacitance=5756.6  Setx0=off  InitialVoltage=0  Measurements=None
  Parallel RLC Branch2 : spsParallelRLCBranchLib/Parallel RLC Branch  LConnTagsString=a  RConnTagsString=__new0  BranchType=R  Resistance=1e9  Inductance=1e-3  SetiL0=off  InitialCurrent=0  Capacitance=5756.6  Setx0=off  InitialVoltage=0  Measurements=None
  Scope2 : Scope
  Scope3 : Scope
  Scope4 : Scope
  Variable Resistor : spsVariableResistorLib/Variable Resistor  Rabsmin=1e-3
      settings: LibrarySourceBlock=sps_lib/Passives/Variable Resistor
  Voltage Measurement1 : spsVoltageMeasurementLib/Voltage Measurement  PhasorSimulation=off  OutputType=Complex  PSBequivalent=0
  XY Graph : Record  FileSettingsInternal="{\"entries\":[{\"content\":{\"excelSettings\":{\"content\":{},\"type\":\"Streamout.ExcelSettings\"}},\"type\":\"Streamout.FileSettingStorage\",\"uuid\":\"119a4515-5b95-4443-a4b9-2a5c5643a809\"}],\"packageUris\":[\"http://schema.mathworks.com/mf0/streamout_blocks/R2020a\"],\"version\":\"1.0\"}"  Layout=[1 1]  SignalsInternal="{\"entries\":[{\"content\":{\"signals\":[{\"content\":{\"blockPath\":[\"bus_as_currentsource_charging_discharging_battery_1/Subsystem15/XY Graph\"],\"dimensions\":[1],\"domain\":\"bus_as_currentsource_charging_discharging_battery_1/Subsystem15/XY Graph\",\"lineColor\":\"#77ac30\",\"port\":1,\"sid\":[\"\"],\"signalID\":251,\"signalName\":\"MATLAB Function2\"},\"type\":\"RecordBlkView.Signal\",\"uuid\":\"b14fbff2-5f4c-450d-99b6-f9f7aac31ab7\"},{\"content\":{\"blockPath\":[\"bus_as_currentsource_charging_discharging_battery_1/Subsystem15/XY Graph\"],\"dimensions\":[1],\"domain\":\"bus_as_currentsource_charging_discharging_battery_1/Subsystem15/XY Graph\",\"lineColor\":\"#4dbeee\",\"port\":2,\"sid\":[\"\"],\"signalID\":255,\"signalName\":\"Voltage Measurement1\"},\"type\":\"RecordBlkView.Signal\",\"uuid\":\"04455955-f925-445b-ba33-95f3507b935f\"}]},\"type\":\"RecordBlkView.InputSignals\",\"uuid\":\"5fb37245-cef3-4ad1-ad6f-aedf567daa45\"}],\"packageUris\":[\"http://schema.mathworks.com/mf0/streamout_blocks/R2020a\"],\"version\":\"1.0\"}"  VisualizationBindings="{\"xyplotplugin\":{\"info\":[{\"series\":[],\"subplotID\":1}]}}"  CompatibilityTag=XY
  powergui1 : spspowerguiLib/powergui  Priority=1  SimulationMode=Discrete  SampleTime=2e-7  frequency=60  Iterations=50  frequencyindice=0  Pbase=100e6  ErrMax=1e-4  UnitsV=kV  UnitsW=MW  buscounter=0  FunctionMessages=off  echomessages=off  EnableUseOfTLC=off  CurrentSourceSwitches=off  DisableSnubberDevices=off  DisableRonSwitches=off  DisableVfSwitches=off  DisplayEquations=off  AutomaticDiscreteSolvers=off  SolverType=Tustin/Backward Euler (TBE)  Interpol=off  ExternalGateDelay=off  methode=off  Ts=100  x0status=blocks  SPID=on  SwTol=0  HookPort=off  NonlinearTolerance=1e-4  nMaxIteration=100  ContinueOnMaxIteration=off  RestoreLinks=warning  ResistiveCurrentMeasurement=off  Frange=[0:2:500]  Ylog=off  Xlog=on  ShowGrid=off  save=off  variable=ZData  structure=0  ZoomFFT=off  StartTime=0.0  cycles=1  DisplayStyle=1  fundamental=60  FreqAxis=off  MaxFrequency=1000  frequencyindicesteady=1  RmsSteady=1  display=off
  + : PMIOPort  Side=Right
  - : PMIOPort  Port=2  Side=Left
  wires:
  Current Measurement/1 -> Goto1/1
  From3/1 -> Scope3/1
  Voltage Measurement1/1 -> XY Graph/2, Scope2/1
  MATLAB Function2/1(SOC) -> Delay/1, XY Graph/1, Scope4/1
  From1/1 -> Integrator/1
  MATLAB Function/1(y) -> Controlled Voltage Source/1
  MATLAB Function1/1(y) -> Variable Resistor/1
  Integrator/1 -> MATLAB Function2/1(u), MATLAB Function/1(u)
  Clock/1 -> MATLAB Function2/2(time), MATLAB Function/2(time)
  MATLAB Function/2(SOC) -> Delay1/1, MATLAB Function1/1(SOC)
  Delay/1 -> MATLAB Function2/3(SOC1)
  Delay1/1 -> MATLAB Function/3(SOC1)
  connections:
  Variable Resistor/RConn1 -- Parallel RLC Branch/LConn1
  Parallel RLC Branch1/RConn1 -- Parallel RLC Branch2/LConn1 -- +/RConn1 -- Voltage Measurement1/LConn1
  Voltage Measurement1/LConn2 -- Parallel RLC Branch2/RConn1 -- -/RConn1 -- Current Measurement/LConn1
  Controlled Voltage Source/RConn1 -- Variable Resistor/LConn1
  Current Measurement/RConn1 -- Controlled Voltage Source/LConn1
  Parallel RLC Branch/RConn1 -- Parallel RLC Branch1/LConn1
